simulink model "net_model_5_nodes_distributed_controllers"  (R2024b)
settings: Solver=FixedStepAuto  StartTime=0.0  StopTime=n_max  FixedStep=1  RelTol=1e-3
values from neighbouring files (symbols this model uses):
  A_ctrl = zeros(n, n, n_of_systems)    [compute_controller_sparse.m]    (also in distributed_sw_stable_ctrl_no_sparse_fast.mat = [0.00195454568338 -0.037655256234 -1.01158174588 -1.64189505)
  A_matrices = A_new    [compute_acc_state_space.m]
  B = B_new(:, :, 9)    [compute_acc_state_space.m]
  B_ctrl = -L_mat    [compute_controller_sparse.m]    (also in distributed_sw_stable_ctrl_no_sparse_fast.mat = [0.998045454317 -0.062441607766 0.0357514431801 1.6418950566)
  C = C_new(:, :, 9)    [compute_acc_state_space.m]
  C_ctrl = J_mat    [compute_controller_sparse.m]    (also in distributed_sw_stable_ctrl_no_sparse_fast.mat = [-0.975830302696 -4.92960999652e-13 -0.212682063947 -5.16220)
  D_ctrl = zeros(m, p, n_of_systems)    [compute_controller_sparse.m]    (also in distributed_sw_stable_ctrl_no_sparse_fast.mat = [0 0 0 0 0 0 0 0 0 0 0 0 ... (450 elements, 5x10x9)])
  n_T_local = 30    [main.m]
  node_1_0 = pi / 180 * [5, 0]'    [main.m]
  node_2_0 = pi / 180 * [-8, 0]'    [main.m]
  node_3_0 = pi / 180 * [2, 0]'    [main.m]
  node_4_0 = pi / 180 * [-8, 0]'    [main.m]
  node_5_0 = pi / 180 * [-3, 0]'    [main.m]
  T_A = [0.410659435681 -0.460542113287 -0.24395006617 -0.0377230432056 -0.150727486653 -0.0781659750949 0.0709437199928 -0.0190547057213 0.0964000848805 0.0445584792865 -0.0447116984993 -0.00701792637604 ... (202500 elements, 150x150x9)]    [T_hinf.mat]    (also in compute_controller_sparse.m = zeros(n_states, n_states, n_of_systems); distributed_sw_stable_ctrl_no_sparse_fast.mat = [0 0 0 0 0 0 0 0 0 0 0 0 ... (225 elements, 5x5x9)]; still_testing_T.m = zeros(5 * n_states, 5 * n_states, n_of_systems))
  T_B = [-24.3939123049 -41.9753912171 83.6712406827 -6.92869753499 -10.2786447385 11.5155106774 58.1276453568 34.021990699 -82.780567 12.8459324222 -18.1653365211 -10.955058798 ... (13500 elements, 150x10x9)]    [T_hinf.mat]    (also in compute_controller_sparse.m = zeros(n_states, 10, n_of_systems); distributed_sw_stable_ctrl_no_sparse_fast.mat = [0 0 0 0 0 0 0 0 0 0 0 0 ... (450 elements, 5x10x9)]; still_testing_T.m = zeros(5 * n_states, 10, n_of_systems))
  T_C = [0.196541617449 0 0 0 0 0.0429189927438 0 0 0 0 0.0856085779401 0 ... (6750 elements, 5x150x9)]    [T_hinf.mat]    (also in compute_controller_sparse.m = zeros(5, n_states, n_of_systems); distributed_sw_stable_ctrl_no_sparse_fast.mat = [0 0 0 0 0 0 0 0 0 0 0 0 ... (225 elements, 5x5x9)]; still_testing_T.m = zeros(5, 5 * n_states, n_of_systems))
  T_D = [7.54968882163 0 0 0 0 3.54430938537 0 0 0 0 0 128.290100624 ... (450 elements, 5x10x9)]    [T_hinf.mat]    (also in compute_controller_sparse.m = zeros(5, 10, n_of_systems); distributed_sw_stable_ctrl_no_sparse_fast.mat = [0 0 0 0 0 0 0 0 0 0 0 0 ... (450 elements, 5x10x9)]; still_testing_T.m = zeros(5, 10, n_of_systems))
undefined symbols (not defined in the file or in its folder): a, Bt, Ct, DiscIntNeverNeededParam
(part 2 of 2)

== system net_model_5_nodes_distributed_controllers/Network Configuration Selector/Node 4 Inputs ==
  Line 4 - 2 : Inport
  Line 4 - 3 : Inport  Port=2
  Line 4 - 5 : Inport  Port=3
  Constant{3,5,7,9..10} (5 alike) : Constant  Value=0
  Constant4 : Constant  Value=0.8433
  Constant6 : Constant  Value=0.8259
  Constant8 : Constant  Value=0.8367
  Mux1 : Mux  Inputs=5
  Switch1 : Switch  Criteria=u2 ~= 0  SaturateOnIntegerOverflow=off  InputSameDT=off
  Switch2 : Switch  Criteria=u2 ~= 0  SaturateOnIntegerOverflow=off  InputSameDT=off
  Switch3 : Switch  Criteria=u2 ~= 0  SaturateOnIntegerOverflow=off  InputSameDT=off
  Out1 : Outport
  wires:
  Mux1/1 -> Out1/1
  Line 4 - 2/1 -> Switch1/2
  Line 4 - 5/1 -> Switch3/2
  Constant5/1 -> Switch1/3
  Switch3/1 -> Mux1/5
  Constant8/1 -> Switch3/1
  Constant9/1 -> Switch3/3
  Constant7/1 -> Switch2/3
  Constant4/1 -> Switch1/1
  Constant6/1 -> Switch2/1
  Line 4 - 3/1 -> Switch2/2
  Constant3/1 -> Mux1/1
  Constant10/1 -> Mux1/4
  Switch2/1 -> Mux1/3
  Switch1/1 -> Mux1/2

== system net_model_5_nodes_distributed_controllers/Network Configuration Selector/Node 4 Inputs1 ==
  Line 5 - 1 : Inport
  Line 5 - 2 : Inport  Port=2
  Line 5 - 3 : Inport  Port=3
  Line 5 - 4 : Inport  Port=4
  Constant1 : Constant  Value=0.7513
  Constant{2..3,5,7,9} (5 alike) : Constant  Value=0
  Constant4 : Constant  Value=0.6318
  Constant6 : Constant  Value=0.8620
  Constant8 : Constant  Value=0.8367
  Mux1 : Mux  Inputs=5
  Switch{1..4} (4 alike) : Switch  Criteria=u2 ~= 0  SaturateOnIntegerOverflow=off  InputSameDT=off
  Out1 : Outport
  wires:
  Line 5 - 2/1 -> Switch1/2
  Switch1/1 -> Mux1/2
  Constant7/1 -> Switch2/3
  Constant6/1 -> Switch2/1
  Constant4/1 -> Switch1/1
  Constant9/1 -> Switch3/3
  Constant8/1 -> Switch3/1
  Line 5 - 3/1 -> Switch2/2
  Line 5 - 4/1 -> Switch3/2
  Mux1/1 -> Out1/1
  Constant5/1 -> Switch1/3
  Switch2/1 -> Mux1/3
  Constant1/1 -> Switch4/1
  Constant2/1 -> Switch4/3
  Switch4/1 -> Mux1/1
  Line 5 - 1/1 -> Switch4/2
  Switch3/1 -> Mux1/4
  Constant3/1 -> Mux1/5

== matlab function net_model_5_nodes_distributed_controllers/Node 5/Interface ==
  data: delta_1 input; neigh_values output; delta_2 input; delta_3 input; delta_4 input; l_5q input
function neigh_values = fcn(delta_1, delta_2, delta_3, delta_4, l_5q)

    neigh_values = l_5q(1) * delta_1 + l_5q(2) * delta_2 + l_5q(3) * delta_3 + l_5q(4) * delta_4;

end

== matlab function net_model_5_nodes_distributed_controllers/Node 5/Node dynamics ==
  data: x_prev input; u input; x output; w input; neigh_values input; l_iq input; current_node input
function x = fcn(x_prev, u, w, neigh_values, l_iq, current_node)
    
    % current_node = 1;

%%

    hi = [0.3244
        1.5886;
        0.6224;
        1.0571;
        0.3313];

    di = [0.5650;
        0.7844;
        0.7347;
        0.5060;
        0.6686];

    dt = 0.2;
%%

    a21 = -hi(current_node) * dt * sum(l_iq);
    a22 = 1 - hi(current_node) * di(current_node) * dt;

    A = [1, dt;
        a21, a22];

    x = A * x_prev + [0 1]' * (u + w + hi(current_node) * dt * neigh_values);
    
end

== matlab function net_model_5_nodes_distributed_controllers/Node 1/Interface ==
  data: delta_2 input; delta_3 input; delta_5 input; neigh_values output; l_1q input
function neigh_values = fcn(delta_2, delta_3, delta_5, l_1q)

    neigh_values = l_1q(2) * delta_2 + l_1q(3) * delta_3 + l_1q(5) * delta_5;

end

== matlab function net_model_5_nodes_distributed_controllers/Node 1/Node dynamics ==
  data: x_prev input; u input; x output; w input; neigh_values input; l_iq input; current_node input
function x = fcn(x_prev, u, w, neigh_values, l_iq, current_node)
    
    % current_node = 1;

%%

    hi = [0.3244
        1.5886;
        0.6224;
        1.0571;
        0.3313];

    di = [0.5650;
        0.7844;
        0.7347;
        0.5060;
        0.6686];

    dt = 0.2;
%%

    a21 = -hi(current_node) * dt * sum(l_iq);
    a22 = 1 - hi(current_node) * di(current_node) * dt;

    A = [1, dt;
        a21, a22];

    x = A * x_prev + [0 1]' * (u + w + hi(current_node) * dt * neigh_values);
    
end

== matlab function net_model_5_nodes_distributed_controllers/Node 3/Interface ==
  data: delta_1 input; neigh_values output; delta_4 input; delta_5 input; l_3q input
function neigh_values = fcn(delta_1, delta_4, delta_5, l_3q)

    neigh_values = l_3q(1) * delta_1 + l_3q(4) * delta_4 + l_3q(5) * delta_5;

end

== matlab function net_model_5_nodes_distributed_controllers/Node 3/Node dynamics ==
  data: x_prev input; u input; x output; w input; neigh_values input; l_iq input; current_node input
function x = fcn(x_prev, u, w, neigh_values, l_iq, current_node)
    
    % current_node = 1;

%%

    hi = [0.3244
        1.5886;
        0.6224;
        1.0571;
        0.3313];

    di = [0.5650;
        0.7844;
        0.7347;
        0.5060;
        0.6686];
    dt = 0.2;
%%

    a21 = -hi(current_node) * dt * sum(l_iq);
    a22 = 1 - hi(current_node) * di(current_node) * dt;

    A = [1, dt;
        a21, a22];

    x = A * x_prev + [0 1]' * (u + w + hi(current_node) * dt * neigh_values);
    
end

== matlab function net_model_5_nodes_distributed_controllers/Node 2/Interface ==
  data: delta_1 input; neigh_values output; delta_4 input; delta_5 input; l_2q input
function neigh_values = fcn(delta_1, delta_4, delta_5, l_2q)

    neigh_values = l_2q(1) * delta_1 + l_2q(4) * delta_4 + l_2q(5) * delta_5;

end

== matlab function net_model_5_nodes_distributed_controllers/Node 2/Node dynamics ==
  data: x_prev input; u input; x output; w input; neigh_values input; l_iq input; current_node input
function x = fcn(x_prev, u, w, neigh_values, l_iq, current_node)
    
    % current_node = 1;

%%

    hi = [0.3244
        1.5886;
        0.6224;
        1.0571;
        0.3313];

    di = [0.5650;
        0.7844;
        0.7347;
        0.5060;
        0.6686];

    dt = 0.2;
%%

    a21 = -hi(current_node) * dt * sum(l_iq);
    a22 = 1 - hi(current_node) * di(current_node) * dt;

    A = [1, dt;
        a21, a22];

    x = A * x_prev + [0 1]' * (u + w + hi(current_node) * dt * neigh_values);
    
end

== matlab function net_model_5_nodes_distributed_controllers/Node 4/Interface ==
  data: delta_2 input; neigh_values output; delta_3 input; delta_5 input; l_4q input
function neigh_values = fcn(delta_2, delta_3, delta_5, l_4q)

    neigh_values = l_4q(2) * delta_2 + l_4q(3) * delta_3 + l_4q(5) * delta_5;

end

== matlab function net_model_5_nodes_distributed_controllers/Node 4/Node dynamics ==
  data: x_prev input; u input; x output; w input; neigh_values input; l_iq input; current_node input
function x = fcn(x_prev, u, w, neigh_values, l_iq, current_node)
    
    % current_node = 1;

%%

    hi = [0.3244
        1.5886;
        0.6224;
        1.0571;
        0.3313];

    di = [0.5650;
        0.7844;
        0.7347;
        0.5060;
        0.6686];

    dt = 0.2;
%%

    a21 = -hi(current_node) * dt * sum(l_iq);
    a22 = 1 - hi(current_node) * di(current_node) * dt;

    A = [1, dt;
        a21, a22];

    x = A * x_prev + [0 1]' * (u + w + hi(current_node) * dt * neigh_values);
    
end
